simulink model "AOs_sim"  (R2022b)
settings: Solver=ode1  StartTime=0.0  StopTime=inf  FixedStep=0.002  RelTol=1e-3
(part 2 of 2)

== system AOs_sim/Knee joint/(2) AOs3/AO4/Φ3_dot(t) ==
  In1 : Inport
  Constant : Constant  Value=3
  Divide : Product  Inputs=*/
  Product : Product  Inputs=3
  Product1 : Product
  Sum : Sum
  cos(Φ(t)) : Fcn  Expr=cos(u(2))
  Φ_dot(t) : Outport
  wires:
  Divide/1 -> Product/2
  Sum/1 -> Φ_dot(t)/1
  In1/1 -> cos(Φ(t))/1
  [vphi_knee] -> Product/1
  cos(Φ(t))/1 -> Product/3
  Product/1 -> Sum/2
  Constant/1 -> Product1/1
  [Omega_knee] -> Product1/2
  Product1/1 -> Sum/1
  [Ft_knee] -> Divide/1
  [SumAlpha_knee] -> Divide/2

== system AOs_sim/Knee joint/(2) AOs3/AO4/α_dot(t) ==
  Input : Inport
  Product : Product  Inputs=3
  sin(Φ3(t)) : Fcn  Expr=sin(u(2))
  α_dot(t) : Outport
  wires:
  Product/1 -> α_dot(t)/1
  [Eta_knee] -> Product/1
  sin(Φ3(t))/1 -> Product/3
  [Ft_knee] -> Product/2
  Input/1 -> sin(Φ3(t))/1

== system AOs_sim/Knee joint/(2) AOs3/AO4/ω_dot(t) ==
  Input : Inport
  Divide : Product  Inputs=*/
  Product : Product  Inputs=3
  cos(Φ1(t)) : Fcn  Expr=cos(u(1))
  ω_dot(t) : Outport
  wires:
  Product/1 -> ω_dot(t)/1
  [vomega_knee] -> Product/1
  Input/1 -> cos(Φ1(t))/1
  cos(Φ1(t))/1 -> Product/3
  [Ft_knee] -> Divide/1
  Divide/1 -> Product/2
  [SumAlpha_knee] -> Divide/2

== system AOs_sim/Knee joint/(3) Phase Error Compensation/Phase Error Calculator/Subsystem ==
  Φn : Inport
  Pe_tilde(tk-1) : Inport  Port=2
  Trigger : TriggerPort  VariantControl=Variant  PortDimensions=1
  PE : Subsystem
  PE Further Updated : Subsystem
  Pe(tk) : Outport
  Pe_tilde(tk) : Outport  Port=2
  wires:
  PE/1(Pe(tk)) -> PE Further Updated/1(Pe(tk)), Pe(tk)/1
  PE Further Updated/1(Pe_tilde(tk)) -> Pe_tilde(tk)/1
  Pe_tilde(tk-1)/1 -> PE Further Updated/2(Pe_tilde(tk-1))
  Φn/1 -> PE/1(Φn(tk))

== system AOs_sim/Knee joint/(3) Phase Error Compensation/Phase Error Calculator/Subsystem1 ==
  Pe_tilde(tk) : Inport
  Trigger : TriggerPort  VariantControl=Variant  PortDimensions=1
  Pe_tilde(tk-1) : Outport
  wires:
  Pe_tilde(tk)/1 -> Pe_tilde(tk-1)/1

== system AOs_sim/Ankle joint/(3) Phase Error Compensation/Phase Error Calculator/Subsystem/PE ==
  Φn(tk) : Inport
  If : If  IfExpression=u1>=0 & u1<3.14
  If Action Subsystem : Subsystem  TreatAsAtomicUnit=on
  If Action Subsystem1 : Subsystem  TreatAsAtomicUnit=on
  Merge : Merge
  Pe(tk) : Outport
  wires:
  Φn(tk)/1 -> If Action Subsystem1/1(Φn(tk)), If Action Subsystem/1(Φn(tk)), If/1
  If/2 -> If Action Subsystem1/Action
  If Action Subsystem/1(Pe(tk)) -> Merge/1
  Merge/1 -> Pe(tk)/1
  If/1 -> If Action Subsystem/Action
  If Action Subsystem1/1(Pe(tk)) -> Merge/2

== system AOs_sim/Ankle joint/(3) Phase Error Compensation/Phase Error Calculator/Subsystem/PE Further Updated ==
  Pe(tk) : Inport
  Pe_tilde(tk-1) : Inport  Port=2
  If : If  NumInputs=2  IfExpression=u1>1.5708 & u2<-1.5708  ElseIfExpressions=u1<-1.5708 & u2>1.5708
  If Action Subsystem : Subsystem  TreatAsAtomicUnit=on
  If Action Subsystem1 : Subsystem  TreatAsAtomicUnit=on
  If Action Subsystem2 : Subsystem  TreatAsAtomicUnit=on
  Merge : Merge  Inputs=3
  Pe_tilde(tk) : Outport
  wires:
  Pe(tk)/1 -> If Action Subsystem2/1(Pe), If Action Subsystem1/1(Pe), If Action Subsystem/1(Pe), If/1
  If/2 -> If Action Subsystem1/Action
  If Action Subsystem/1(Pe_tilde) -> Merge/1
  Merge/1 -> Pe_tilde(tk)/1
  If/1 -> If Action Subsystem/Action
  If Action Subsystem1/1(Pe_tilde) -> Merge/2
  If/3 -> If Action Subsystem2/Action
  If Action Subsystem2/1(Pe_tilde) -> Merge/3
  Pe_tilde(tk-1)/1 -> If/2

== system AOs_sim/Hip joint/(3) Phase Error Compensation/Phase Error Calculator/Subsystem/PE ==
  Φn(tk) : Inport
  If : If  IfExpression=u1>=0 & u1<3.14
  If Action Subsystem : Subsystem  TreatAsAtomicUnit=on
  If Action Subsystem1 : Subsystem  TreatAsAtomicUnit=on
  Merge : Merge
  Pe(tk) : Outport
  wires:
  Φn(tk)/1 -> If Action Subsystem1/1(Φn(tk)), If Action Subsystem/1(Φn(tk)), If/1
  If/2 -> If Action Subsystem1/Action
  If Action Subsystem/1(Pe(tk)) -> Merge/1
  Merge/1 -> Pe(tk)/1
  If/1 -> If Action Subsystem/Action
  If Action Subsystem1/1(Pe(tk)) -> Merge/2

== system AOs_sim/Hip joint/(3) Phase Error Compensation/Phase Error Calculator/Subsystem/PE Further Updated ==
  Pe(tk) : Inport
  Pe_tilde(tk-1) : Inport  Port=2
  If : If  NumInputs=2  IfExpression=u1>1.5708 & u2<-1.5708  ElseIfExpressions=u1<-1.5708 & u2>1.5708
  If Action Subsystem : Subsystem  TreatAsAtomicUnit=on
  If Action Subsystem1 : Subsystem  TreatAsAtomicUnit=on
  If Action Subsystem2 : Subsystem  TreatAsAtomicUnit=on
  Merge : Merge  Inputs=3
  Pe_tilde(tk) : Outport
  wires:
  Pe(tk)/1 -> If Action Subsystem2/1(Pe), If Action Subsystem1/1(Pe), If Action Subsystem/1(Pe), If/1
  If/2 -> If Action Subsystem1/Action
  If Action Subsystem/1(Pe_tilde) -> Merge/1
  Merge/1 -> Pe_tilde(tk)/1
  If/1 -> If Action Subsystem/Action
  If Action Subsystem1/1(Pe_tilde) -> Merge/2
  If/3 -> If Action Subsystem2/Action
  If Action Subsystem2/1(Pe_tilde) -> Merge/3
  Pe_tilde(tk-1)/1 -> If/2

== system AOs_sim/Knee joint/(3) Phase Error Compensation/Phase Error Calculator/Subsystem/PE ==
  Φn(tk) : Inport
  If : If  IfExpression=u1>=0 & u1<3.14
  If Action Subsystem : Subsystem  TreatAsAtomicUnit=on
  If Action Subsystem1 : Subsystem  TreatAsAtomicUnit=on
  Merge : Merge
  Pe(tk) : Outport
  wires:
  Φn(tk)/1 -> If Action Subsystem1/1(Φn(tk)), If Action Subsystem/1(Φn(tk)), If/1
  If/2 -> If Action Subsystem1/Action
  If Action Subsystem/1(Pe(tk)) -> Merge/1
  Merge/1 -> Pe(tk)/1
  If/1 -> If Action Subsystem/Action
  If Action Subsystem1/1(Pe(tk)) -> Merge/2

== system AOs_sim/Knee joint/(3) Phase Error Compensation/Phase Error Calculator/Subsystem/PE Further Updated ==
  Pe(tk) : Inport
  Pe_tilde(tk-1) : Inport  Port=2
  If : If  NumInputs=2  IfExpression=u1>1.5708 & u2<-1.5708  ElseIfExpressions=u1<-1.5708 & u2>1.5708
  If Action Subsystem : Subsystem  TreatAsAtomicUnit=on
  If Action Subsystem1 : Subsystem  TreatAsAtomicUnit=on
  If Action Subsystem2 : Subsystem  TreatAsAtomicUnit=on
  Merge : Merge  Inputs=3
  Pe_tilde(tk) : Outport
  wires:
  Pe(tk)/1 -> If Action Subsystem2/1(Pe), If Action Subsystem1/1(Pe), If Action Subsystem/1(Pe), If/1
  If/2 -> If Action Subsystem1/Action
  If Action Subsystem/1(Pe_tilde) -> Merge/1
  Merge/1 -> Pe_tilde(tk)/1
  If/1 -> If Action Subsystem/Action
  If Action Subsystem1/1(Pe_tilde) -> Merge/2
  If/3 -> If Action Subsystem2/Action
  If Action Subsystem2/1(Pe_tilde) -> Merge/3
  Pe_tilde(tk-1)/1 -> If/2

== system AOs_sim/Ankle joint/(3) Phase Error Compensation/Phase Error Calculator/Subsystem/PE/If Action Subsystem ==
  Φn(tk) : Inport
  Action Port : ActionPort  ActionPortLabel=if(u1>=0 & u1<3.14)
  Gain : Gain  Gain=-1
  Pe(tk) : Outport
  wires:
  Gain/1 -> Pe(tk)/1
  Φn(tk)/1 -> Gain/1

== system AOs_sim/Ankle joint/(3) Phase Error Compensation/Phase Error Calculator/Subsystem/PE/If Action Subsystem1 ==
  Φn(tk) : Inport
  Action Port : ActionPort  ActionPortLabel=else
  Constant : Constant  Value=2*pi
  Minus : Sum  Inputs=-+
  Pe(tk) : Outport
  wires:
  Constant/1 -> Minus/2
  Minus/1 -> Pe(tk)/1
  Φn(tk)/1 -> Minus/1

== system AOs_sim/Ankle joint/(3) Phase Error Compensation/Phase Error Calculator/Subsystem/PE Further Updated/If Action Subsystem ==
  Pe : Inport
  Action Port : ActionPort  ActionPortLabel=if(u1>1.5708 & u2<-1.5708)
  Constant : Constant  Value=2*pi
  Minus : Sum  Inputs=+-
  Pe_tilde : Outport
  wires:
  Constant/1 -> Minus/2
  Minus/1 -> Pe_tilde/1
  Pe/1 -> Minus/1

== system AOs_sim/Ankle joint/(3) Phase Error Compensation/Phase Error Calculator/Subsystem/PE Further Updated/If Action Subsystem1 ==
  Pe : Inport
  Action Port : ActionPort  ActionPortLabel=elseif(u1<-1.5708 & u2>1.5708)
  Constant : Constant  Value=2*pi
  Minus : Sum
  Pe_tilde : Outport
  wires:
  Constant/1 -> Minus/2
  Minus/1 -> Pe_tilde/1
  Pe/1 -> Minus/1

== system AOs_sim/Ankle joint/(3) Phase Error Compensation/Phase Error Calculator/Subsystem/PE Further Updated/If Action Subsystem2 ==
  Pe : Inport
  Action Port : ActionPort  ActionPortLabel=else
  Pe_tilde : Outport
  wires:
  Pe/1 -> Pe_tilde/1

== system AOs_sim/Hip joint/(3) Phase Error Compensation/Phase Error Calculator/Subsystem/PE/If Action Subsystem ==
  Φn(tk) : Inport
  Action Port : ActionPort  ActionPortLabel=if(u1>=0 & u1<3.14)
  Gain : Gain  Gain=-1
  Pe(tk) : Outport
  wires:
  Gain/1 -> Pe(tk)/1
  Φn(tk)/1 -> Gain/1

== system AOs_sim/Hip joint/(3) Phase Error Compensation/Phase Error Calculator/Subsystem/PE/If Action Subsystem1 ==
  Φn(tk) : Inport
  Action Port : ActionPort  ActionPortLabel=else
  Constant : Constant  Value=2*pi
  Minus : Sum  Inputs=-+
  Pe(tk) : Outport
  wires:
  Constant/1 -> Minus/2
  Minus/1 -> Pe(tk)/1
  Φn(tk)/1 -> Minus/1

== system AOs_sim/Hip joint/(3) Phase Error Compensation/Phase Error Calculator/Subsystem/PE Further Updated/If Action Subsystem ==
  Pe : Inport
  Action Port : ActionPort  ActionPortLabel=if(u1>1.5708 & u2<-1.5708)
  Constant : Constant  Value=2*pi
  Minus : Sum  Inputs=+-
  Pe_tilde : Outport
  wires:
  Constant/1 -> Minus/2
  Minus/1 -> Pe_tilde/1
  Pe/1 -> Minus/1

== system AOs_sim/Hip joint/(3) Phase Error Compensation/Phase Error Calculator/Subsystem/PE Further Updated/If Action Subsystem1 ==
  Pe : Inport
  Action Port : ActionPort  ActionPortLabel=elseif(u1<-1.5708 & u2>1.5708)
  Constant : Constant  Value=2*pi
  Minus : Sum
  Pe_tilde : Outport
  wires:
  Constant/1 -> Minus/2
  Minus/1 -> Pe_tilde/1
  Pe/1 -> Minus/1

== system AOs_sim/Hip joint/(3) Phase Error Compensation/Phase Error Calculator/Subsystem/PE Further Updated/If Action Subsystem2 ==
  Pe : Inport
  Action Port : ActionPort  ActionPortLabel=else
  Pe_tilde : Outport
  wires:
  Pe/1 -> Pe_tilde/1

== system AOs_sim/Knee joint/(3) Phase Error Compensation/Phase Error Calculator/Subsystem/PE/If Action Subsystem ==
  Φn(tk) : Inport
  Action Port : ActionPort  ActionPortLabel=if(u1>=0 & u1<3.14)
  Gain : Gain  Gain=-1
  Pe(tk) : Outport
  wires:
  Gain/1 -> Pe(tk)/1
  Φn(tk)/1 -> Gain/1

== system AOs_sim/Knee joint/(3) Phase Error Compensation/Phase Error Calculator/Subsystem/PE/If Action Subsystem1 ==
  Φn(tk) : Inport
  Action Port : ActionPort  ActionPortLabel=else
  Constant : Constant  Value=2*pi
  Minus : Sum  Inputs=-+
  Pe(tk) : Outport
  wires:
  Constant/1 -> Minus/2
  Minus/1 -> Pe(tk)/1
  Φn(tk)/1 -> Minus/1

== system AOs_sim/Knee joint/(3) Phase Error Compensation/Phase Error Calculator/Subsystem/PE Further Updated/If Action Subsystem ==
  Pe : Inport
  Action Port : ActionPort  ActionPortLabel=if(u1>1.5708 & u2<-1.5708)
  Constant : Constant  Value=2*pi
  Minus : Sum  Inputs=+-
  Pe_tilde : Outport
  wires:
  Constant/1 -> Minus/2
  Minus/1 -> Pe_tilde/1
  Pe/1 -> Minus/1

== system AOs_sim/Knee joint/(3) Phase Error Compensation/Phase Error Calculator/Subsystem/PE Further Updated/If Action Subsystem1 ==
  Pe : Inport
  Action Port : ActionPort  ActionPortLabel=elseif(u1<-1.5708 & u2>1.5708)
  Constant : Constant  Value=2*pi
  Minus : Sum
  Pe_tilde : Outport
  wires:
  Constant/1 -> Minus/2
  Minus/1 -> Pe_tilde/1
  Pe/1 -> Minus/1

== system AOs_sim/Knee joint/(3) Phase Error Compensation/Phase Error Calculator/Subsystem/PE Further Updated/If Action Subsystem2 ==
  Pe : Inport
  Action Port : ActionPort  ActionPortLabel=else
  Pe_tilde : Outport
  wires:
  Pe/1 -> Pe_tilde/1
